simulink model "encoder_conv"  (R2025b)
settings: Solver=FixedStepAuto  StartTime=0.0  StopTime=inf  RelTol=1e-3
libraries: commcnvcod2 x2, commdigbbndpm3 x1, commrandsrc3 x1, commsink2 x1
settings Model: Creator=briyi  LastModifiedBy=briyi

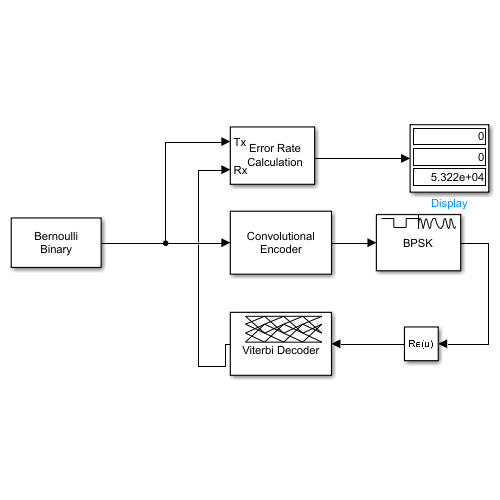
[thumbnail: Simulink's stored preview of the top-level diagram]
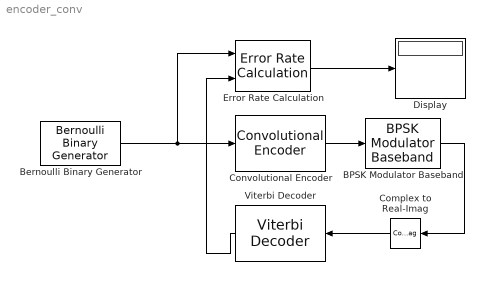
== system encoder_conv ==
  BPSK Modulator Baseband : commdigbbndpm3/BPSK Modulator Baseband  Ph=0  outDtype=double  outWordLen=16  outUDDataType=sfix(16)  outFracLenMode=Best precision  outFracLen=15  outDataTypeStr=double  outLastDataTypeStr=double
  Bernoulli Binary Generator : commrandsrc3/Bernoulli Binary Generator  ProbabilityOfZero=0.5  SeedSource=Parameter  Seed=61  SampleTime=1  SamplesPerFrame=1  OutputDataType=double  SimulateUsing=Interpreted execution
  Complex to Real-Imag : ComplexToRealImag  Output=Real
  Convolutional Encoder : commcnvcod2/Convolutional Encoder  trellis=poly2trellis(7, [171 133])  opMode=Continuous  DelayedResetAction=off  hasIniStPort=off  hasFinStPort=off  usePuncVector=off  punctureVector=[1; 1; 0; 1; 0; 1]  reset=Unused parameter value
  Display : Display
  Error Rate Calculation : commsink2/Error Rate Calculation  N=96  st_delay=0  cp_mode=Entire frame  subframe=[]  PMode=Port  WsName=ErrorVec  RsMode2=off  stop=off  numErr=100  maxBits=1e6
  Viterbi Decoder : commcnvcod2/Viterbi Decoder  trellis=poly2trellis(7,[171 133])  isPunctured=off  punctureVector=[1; 1; 0; 1; 0; 1]  erasures=off  dectype=Unquantized  nsdecb=3  runSigValErrCheck=off  tbdepth=96  opmode=Continuous  reset=off  delayedResetAction=off  smWordLength=16  outDataType=Inherit via internal rule
  wires:
  Bernoulli Binary Generator/1 -> Error Rate Calculation/1, Convolutional Encoder/1
  Viterbi Decoder/1 -> Error Rate Calculation/2
  Error Rate Calculation/1 -> Display/1
  Convolutional Encoder/1 -> BPSK Modulator Baseband/1
  BPSK Modulator Baseband/1 -> Complex to Real-Imag/1
  Complex to Real-Imag/1 -> Viterbi Decoder/1
